simulink model "controller"  (R2014a)
settings: Solver=ode3  StartTime=0.0  StopTime=300  FixedStep=0.01  RelTol=1e-3
values from neighbouring files (symbols this model uses):
  D0 = 10    [Modified_Bergman.m]
  drate = 0.05    [Modified_Bergman.m]
  G0 = Gb + p0    (= 276)    [Modified_Bergman.m]    (also in data.m = 287)
  G_set = 150    [Modified_Bergman.m]
  Gb = 81    [Modified_Bergman.m]    (also in data.m = 92)
  I0 = Ib + 396    (= 411)    [Modified_Bergman.m]    (also in data.m = 300)
  Ib = 15    [Modified_Bergman.m]    (also in data.m = 7.3)
  p1 = 0.028735    [Modified_Bergman.m]    (also in data.m = 0.03082)
  p2 = 0.028344    [Modified_Bergman.m]    (also in data.m = 0.02093)
  p3 = 5.035E-5    (= 5.035e-05)    [Modified_Bergman.m]    (also in data.m = 1.06e-05)
  p4 = 0.3    [Modified_Bergman.m]    (also in data.m)
  Rultn = 0.74    [Modified_Bergman.m]
  X0 = 0    [Modified_Bergman.m]    (also in data.m)
libraries: simulink x2
settings Model: Creator=sameer  LastModifiedBy=sameer

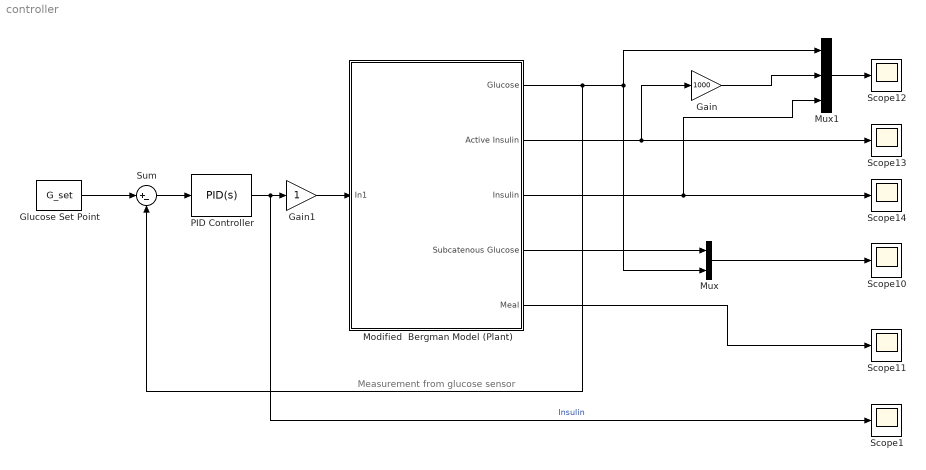
== system controller ==
  note: Measurement from glucose sensor
  Gain : Gain  Gain=1000
  Gain1 : Gain
  Glucose Set Point : Constant  Value=G_set
  "Modified  Bergman Model (Plant) " : Subsystem
  Mux : Mux  Inputs=2
  Mux1 : Mux  Inputs=3
  PID Controller : simulink/Continuous/PID Controller  Controller=PID  TimeDomain=Continuous-time  SampleTime=1  IntegratorMethod=Forward Euler  FilterMethod=Forward Euler  Form=Parallel  P=-0.0799174114933091  I=-0.00108093836895816  D=-1.45148337052854  N=7.47667341276185  InitialConditionSource=internal  InitialConditionForIntegrator=0  InitialConditionForFilter=0  ExternalReset=none  LimitOutput=on  UpperSaturationLimit=200  LowerSaturationLimit=0  LinearizeAsGain=off  AntiWindupMode=none  Kb=1  TrackingMode=off  Kt=1  PParamMin=[]  PParamMax=[]  IParamMin=[]  IParamMax=[]  DParamMin=[]  DParamMax=[]  NParamMin=[]  NParamMax=[]  KbParamMin=[]  KbParamMax=[]  KtParamMin=[]  KtParamMax=[]  POutMin=[]  POutMax=[]  IOutMin=[]  IOutMax=[]  DOutMin=[]  DOutMax=[]  NOutMin=[]  NOutMax=[]  KbOutMin=[]  KbOutMax=[]  KtOutMin=[]  KtOutMax=[]  IntegratorOutMin=[]  IntegratorOutMax=[]  FilterOutMin=[]  FilterOutMax=[]  SumOutMin=[]  SumOutMax=[]  SumI1OutMin=[]  SumI1OutMax=[]  SumI2OutMin=[]  SumI2OutMax=[]  SumI3OutMin=[]  SumI3OutMax=[]  SumDOutMin=[]  SumDOutMax=[]  SaturationOutMin=[]  SaturationOutMax=[]  IntegratorContinuousStateAttributes=''  IntegratorStateMustResolveToSignalObject=off  IntegratorRTWStateStorageClass=Auto  FilterContinuousStateAttributes=''  FilterStateMustResolveToSignalObject=off  FilterRTWStateStorageClass=Auto
  Scope{1,10..14} (6 alike) : Scope
      Scope1 settings: ShowLegends=on  SaveName=Meal1
      Scope10 settings: ShowLegends=on  TimeRange=100  SaveName=Gsc
      Scope11 settings: ShowLegends=on  SaveName=Meal
      Scope12 settings: ShowLegends=on  TimeRange=500  YMin=-100  YMax=14000000000000  SaveName=Data
      Scope13 settings: ShowLegends=on  SaveName=Active_Insulin
      Scope14 settings: ShowLegends=on  SaveName=Insulin
  Sum : Sum  Inputs=|+-
  wires:
  Sum/1 -> PID Controller/1
  Glucose Set Point/1 -> Sum/1
  "Modified  Bergman Model (Plant) "/1(Glucose) -> Sum/2, Mux/2, Mux1/1
  "Modified  Bergman Model (Plant) "/2(Active Insulin) -> Gain/1, Scope13/1
  "Modified  Bergman Model (Plant) "/3(Insulin) -> Scope14/1, Mux1/3
  "Modified  Bergman Model (Plant) "/4(Subcatenous Glucose) -> Mux/1
  Mux/1 -> Scope10/1
  "Modified  Bergman Model (Plant) "/5(Meal) -> Scope11/1
  Mux1/1 -> Scope12/1
  Gain/1 -> Mux1/2
  PID Controller/1 -> Scope1/1, Gain1/1  "Insulin"
  Gain1/1 -> "Modified  Bergman Model (Plant) "/1(In1)

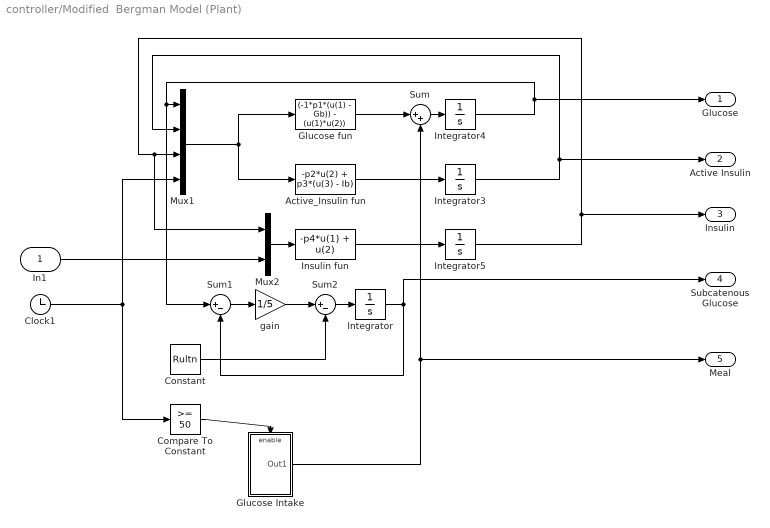
== system controller/Modified  Bergman Model (Plant)  ==
  In1 : Inport
  Active_Insulin fun : Fcn  Expr=-p2*u(2) + p3*(u(3) - Ib)
  Clock1 : Clock
  Compare To Constant : simulink/Logic and Bit Operations/Compare To Constant  relop=>=  const=50  OutDataTypeStr=boolean
  Constant : Constant  Value=Rultn
  Glucose fun : Fcn  Expr=(-1*p1*(u(1) - Gb)) - (u(1)*u(2))
  "Glucose Intake " : Subsystem
  Insulin fun : Fcn  Expr=-p4*u(1) + u(2)
  Integrator : Integrator  InitialCondition=G0 - 5*Rultn
  Integrator3 : Integrator  InitialCondition=X0
  Integrator4 : Integrator  InitialCondition=G0
  Integrator5 : Integrator  InitialCondition=I0
  Mux1 : Mux
  Mux2 : Mux  Inputs=2
  Sum : Sum  Inputs=|++
  Sum1 : Sum  Inputs=|+-
  Sum2 : Sum  Inputs=|+-
  gain : Gain  Gain=1/5
  Glucose : Outport
  Active Insulin : Outport  Port=2
  Insulin : Outport  Port=3
  Subcatenous Glucose : Outport  Port=4
  Meal : Outport  Port=5
  wires:
  gain/1 -> Sum2/1
  Constant/1 -> Sum2/2
  Sum1/1 -> gain/1
  Sum2/1 -> Integrator/1
  Integrator/1 -> Sum1/2, Subcatenous Glucose/1
  In1/1 -> Mux2/2
  Mux2/1 -> Insulin fun/1
  Insulin fun/1 -> Integrator5/1
  Integrator4/1 -> Glucose/1, Mux1/1, Sum1/1
  Glucose fun/1 -> Sum/1
  Integrator5/1 -> Insulin/1, Mux2/1, Mux1/3
  Mux1/1 -> Active_Insulin fun/1, Glucose fun/1
  Active_Insulin fun/1 -> Integrator3/1
  Sum/1 -> Integrator4/1
  Clock1/1 -> Compare To Constant/1, Mux1/4
  Compare To Constant/1 -> "Glucose Intake "/Enable
  Integrator3/1 -> Active Insulin/1, Mux1/2
  "Glucose Intake "/1(Out1) -> Sum/2, Meal/1

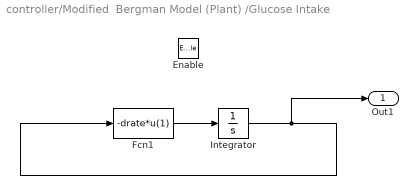
== system controller/Modified  Bergman Model (Plant) /Glucose Intake  ==
  Enable : EnablePort
  Fcn1 : Fcn  Expr=-drate*u(1)
  Integrator : Integrator  InitialCondition=D0
  Out1 : Outport
  wires:
  Integrator/1 -> Fcn1/1, Out1/1
  Fcn1/1 -> Integrator/1
